simulink model "model_simulink"  (Simulink 8.5)
settings: Solver=ode45  StartTime=0.0  StopTime=0.001  RelTol=1e-3
undefined symbols (not defined in the file): C, K, R1, R2, T
settings Model: Creator=Daniel Santos  LastModifiedBy=Daniel Santos
settings DataIOCC: SignalLoggingSaveFormat=Dataset
settings OptimizationCC: ExpressionDepthLimit=128
settings DebuggingCC: UnderspecifiedInitializationDetection=Simplified  MergeDetectMultiDrivingBlocksExec=error  FcnCallInpInsideContextMsg=EnableAllAsError  StateNameClashWarn=none
settings GRTTargetCC: CombineOutputUpdateFcns=on  GRTInterface=off

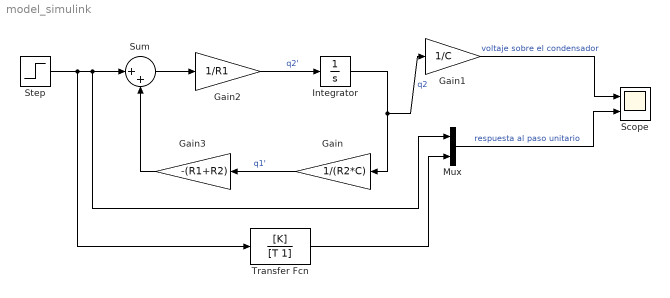
== system model_simulink ==
  Gain : Gain  Gain=1/(R2*C)
  Gain1 : Gain  Gain=1/C
  Gain2 : Gain  Gain=1/R1
  Gain3 : Gain  Gain=-(R1+R2)
  Integrator : Integrator
  Mux : Mux  Inputs=3
  Scope : Scope  NumInputPorts=2
      settings: YMin=-5~-5  YMax=5~5
  Step : Step  Time=0  SampleTime=0
  Sum : Sum  Inputs=|++
  Transfer Fcn : TransferFcn  Numerator=[K]  Denominator=[T 1]
  wires:
  Gain2/1 -> Integrator/1  "q2'"
  Sum/1 -> Gain2/1
  Gain/1 -> Gain3/1  "q1'"
  Gain3/1 -> Sum/2
  Integrator/1 -> Gain/1, Gain1/1  "q2"
  Gain1/1 -> Scope/1  "voltaje sobre el condensador"
  Mux/1 -> Scope/2  "respuesta al paso unitario"
  Step/1 -> Transfer Fcn/1, Mux/1, Sum/1
  Transfer Fcn/1 -> Mux/3
